simulink model "simulador"  (R2012b)
settings: Solver=ode45  StartTime=0.0  StopTime=1  RelTol=1e-6
undefined symbols (not defined in the file): A, B, C, D
settings Model: Creator=Juliano  LastModifiedBy=Juliano

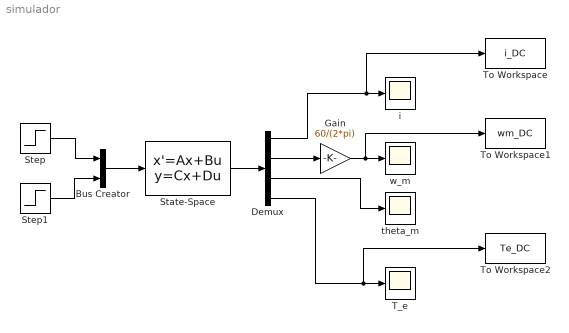
== system simulador ==
  Bus Creator : BusCreator  Inputs=2
  Demux : Demux
  Gain : Gain  Gain=60/(2*pi)
  State-Space : StateSpace  A=A  B=B  C=C  D=D
  Step : Step  Time=0  After=12  SampleTime=0
  Step1 : Step  Time=0.2  After=0*2e-3  SampleTime=0
  T_e : Scope
      settings: SaveName=ScopeData3
  To Workspace : ToWorkspace  VariableName=i_DC  SampleTime=-1  SaveFormat=Timeseries
  To Workspace1 : ToWorkspace  VariableName=wm_DC  SampleTime=-1  SaveFormat=Timeseries
  To Workspace2 : ToWorkspace  VariableName=Te_DC  SampleTime=-1  SaveFormat=Timeseries
  i : Scope
  theta_m : Scope
  w_m : Scope
      settings: YMin=0.21  YMax=0.35  SaveName=ScopeData2
  wires:
  Step/1 -> Bus Creator/1
  Step1/1 -> Bus Creator/2
  Bus Creator/1 -> State-Space/1
  State-Space/1 -> Demux/1
  Demux/3 -> theta_m/1
  Demux/1 -> To Workspace/1, i/1
  Demux/2 -> Gain/1
  Demux/4 -> To Workspace2/1, T_e/1
  Gain/1 -> To Workspace1/1, w_m/1
